simulink model "wheelModel"  (R2020b)
settings: Solver=VariableStepAuto  StartTime=0.0  StopTime=4  RelTol=1e-3
values from neighbouring files (symbols this model uses):
  mass = 1    [editvars.m]    (also in rovervars.mat)
  radius = 0.3    [editvars.m]    (also in rovervars.mat)
  stepTime = 2    [editvars.m]    (also in rovervars.mat)
  torqueF = 0.05    [editvars.m]    (also in rovervars.mat)
settings Model: Creator=lemck  LastModifiedBy=lemck

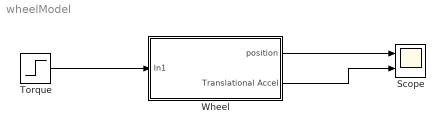
== system wheelModel ==
  Scope : Scope  NumInputPorts=2
  Torque : Step  Time=stepTime  After=torqueF  SampleTime=0
  Wheel : Subsystem
  wires:
  Torque/1 -> Wheel/1(In1)
  Wheel/1(position) -> Scope/1
  Wheel/2(Translational Accel) -> Scope/2

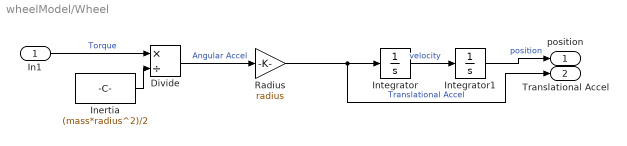
== system wheelModel/Wheel ==
  In1 : Inport
  Divide : Product  Inputs=*/
  Inertia : Constant  Value=(mass*radius^2)/2
  Integrator : Integrator
  Integrator1 : Integrator
  Radius : Gain  Gain=radius
  position : Outport
  Translational Accel : Outport  Port=2
  wires:
  Divide/1 -> Radius/1  "Angular Accel"
  Inertia/1 -> Divide/2
  Integrator/1 -> Integrator1/1  "velocity"
  Radius/1 -> Translational Accel/1, Integrator/1  "Translational Accel"
  In1/1 -> Divide/1  "Torque"
  Integrator1/1 -> position/1  "position"
